simulink model "ToApp"  (R2025b)
settings: Solver=FixedStepDiscrete  StartTime=0.0  StopTime=10.0  FixedStep=0.02  RelTol=1e-3
libraries: dspstat3 x1
settings Model: Creator=Huawei  LastModifiedBy=lolve
settings OptimizationCC: BlockReduction=off  UseDivisionForNetSlopeComputation=on  OptimizeBlockIOStorage=off

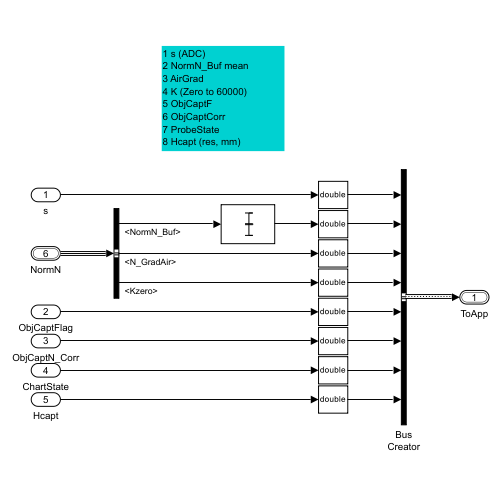
[thumbnail: Simulink's stored preview of the top-level diagram]
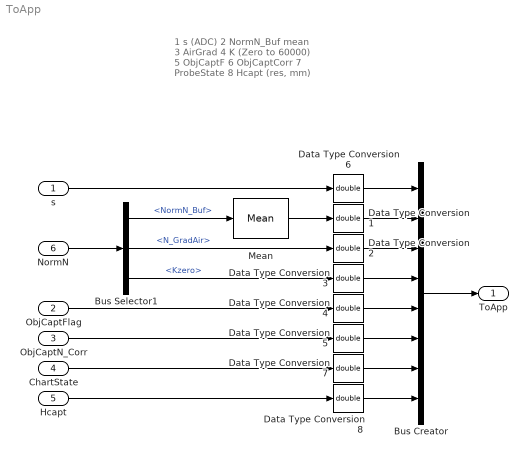
== system ToApp ==
  note: 1 s (ADC)
      | 2 NormN_Buf mean
      | 3 AirGrad
      | 4 K (Zero to 60000)
      | 5 ObjCaptF
      | 6 ObjCaptCorr
      | 7 ProbeState
      | 8 Hcapt (res, mm)
  s : Inport  OutDataTypeStr=uint16  PortDimensions=5000
  ObjCaptFlag : Inport  Port=2  OutDataTypeStr=boolean  PortDimensions=1
  ObjCaptN_Corr : Inport  Port=3  OutDataTypeStr=double  PortDimensions=1
  ChartState : Inport  Port=4  OutDataTypeStr=double  PortDimensions=1
  Hcapt : Inport  Port=5  OutDataTypeStr=double  PortDimensions=1
  NormN : Inport  Port=6  OutDataTypeStr=Bus: N_Bus_Type  PortDimensions=1
  Bus Creator : BusCreator  Inputs=8  OutDataTypeStr=Bus: ToAppBus_Type  NonVirtualBus=on
      settings: InheritFromInputs=off
  Bus Selector1 : BusSelector  OutputSignals=NormN_Buf,N_GradAir,Kzero
  Data Type Conversion{1..8} (8 alike) : DataTypeConversion  OutDataTypeStr=double  SaturateOnIntegerOverflow=off  RndMeth=Floor
  Mean : dspstat3/Mean  run=off  InputProcessing=Columns as channels (frame based)  reset_popup=None  directionMode=Each column  dimension=1  roiEnable=off  roiType=Rectangles  roiPortion=Entire ROI  roiOutput=Individual statistics for each ROI  roiFlag=off  roundingMode=Floor  overflowMode=off  outputDataTypeStr=Inherit: Same as accumulator  outputMin=[]  outputMax=[]  outputLastDataTypeStr=Inherit: Same as accumulator
  ToApp : Outport  OutDataTypeStr=Bus: ToAppBus_Type  BusOutputAsStruct=on
  wires:
  s/1 -> Data Type Conversion6/1
  Hcapt/1 -> Data Type Conversion8/1
  Data Type Conversion8/1 -> Bus Creator/8
  Data Type Conversion4/1 -> Bus Creator/5
  Data Type Conversion2/1 -> Bus Creator/3
  ObjCaptFlag/1 -> Data Type Conversion4/1
  Data Type Conversion1/1 -> Bus Creator/2
  Data Type Conversion3/1 -> Bus Creator/4
  ObjCaptN_Corr/1 -> Data Type Conversion5/1
  Bus Selector1/2 -> Data Type Conversion2/1  "<N_GradAir>"
  Data Type Conversion7/1 -> Bus Creator/7
  Data Type Conversion5/1 -> Bus Creator/6
  Bus Selector1/1 -> Mean/1  "<NormN_Buf>"
  Bus Selector1/3 -> Data Type Conversion3/1  "<Kzero>"
  Mean/1 -> Data Type Conversion1/1
  NormN/1 -> Bus Selector1/1
  ChartState/1 -> Data Type Conversion7/1
  Bus Creator/1 -> ToApp/1
  Data Type Conversion6/1 -> Bus Creator/1
